simulink model "combined"  (R2013a)
settings: Solver=ode45  StartTime=0.0  StopTime=10.0  RelTol=1e-3
settings Model: Creator=eiseles  LastModifiedBy=eiseles

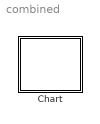
== system combined ==
  Chart : Stateflow chart  TreatAsAtomicUnit=on

== stateflow chart combined/Chart ==
  state PC [parallel]
    settings: executionOrder=2
  state Dongle [parallel]
    settings: executionOrder=3
  state Robot [parallel]
    settings: executionOrder=1
    state Ready
    state Convert
    state Send_wait
      en: i++;
    state Error
    Ready -> Convert : after(200, msec)
    (default) -> Ready
    Send_wait -> Ready [order 3] : [ackDon ==1]
    Convert -> Send_wait : after(3, msec)
    Send_wait -> Error [order 2] : [i>=5]
    Send_wait -> Send_wait [order 1] : after(1, sec)
  data: i local double =0
